simulink model "ap_12BAdapted"  (R2019b)
settings: Solver=FixedStepDiscrete  StartTime=0.0  StopTime=500  FixedStep=Ts  RelTol=1e-3  EnableMultiTasking=on
undefined symbols (not defined in the file): beaver_b, beaver_c, beaver_mass, beaver_S, Cl0, Cl_alpha2_dpt, Cl_beta, Cl_da, Cl_da_alpha, Cl_dr, Cl_p, Cl_r, Cm0, Cm_alpha, Cm_alpha2, Cm_beta2, Cm_de, Cm_df, Cm_dpt, Cm_q, Cm_r, Cn0, Cn_beta, Cn_beta3, Cn_da, Cn_dpt3, Cn_dr, Cn_p, Cn_q, Cn_r, Cx0, Cx_alpha, Cx_alpha2, Cx_alpha3, Cx_df, Cx_df_alpha, Cx_dpt, Cx_dpt2_alpha, Cx_dr, Cx_q, Cy0, Cy_beta, Cy_da, Cy_dr, Cy_dr_alpha, Cy_p, Cy_r, Cz0, Cz_alpha, Cz_alpha3, Cz_de, Cz_de_beta, Cz_df, Cz_df_alpha, Cz_dpt, Cz_q, d2r, fin_act_1, fin_act_2, fin_act_3 ... (+23)
libraries: simulink x10
(part 1 of 3)
settings Model: Creator=elliocm  LastModifiedBy=hbourbou
settings DataIOCC: LimitDataPoints=on  SaveFormat=Array  ReturnWorkspaceOutputs=off
settings OptimizationCC: ExpressionDepthLimit=2147483647  LifeSpan=inf
settings DebuggingCC: SolverPrmCheckMsg=warning  StateNameClashWarn=warning  SFUnexpectedBacktrackingDiag=warning  SFNoUnconditionalDefaultTransitionDiag=warning  SFExecutionAtInitializationDiag=none  ArithmeticOperatorsInVariantConditions=warning
settings HardwareCC: ProdBitPerPointer=32  ProdBitPerSizeT=32  ProdBitPerPtrDiffT=32  ProdLargestAtomicFloat=None  ProdIntDivRoundTo=Undefined  ProdEndianess=Unspecified  ProdWordSize=32  ProdHWDeviceType=32-bit Generic
settings ModelReferenceCC: PropagateSignalLabelsOutOfModel=off
settings SFSimCC: SimUseLocalCustomCode=off  CustomCodeUndefinedFunction=UseInterfaceOnly
settings RTWCC: RTWUseLocalCustomCode=off
settings CodeAppCC: StateflowObjectComments=on
settings GRTTargetCC: TargetLangStandard=C89/C90 (ANSI)  GeneratePreprocessorConditionals=Disable all
settings ConfigComp: CovMetricSettings=dw  CovHtmlReporting=on  CovSaveCumulativeToWorkspaceVar=on  CovSaveSingleToWorkspaceVar=on  CovExternalEMLEnable=off

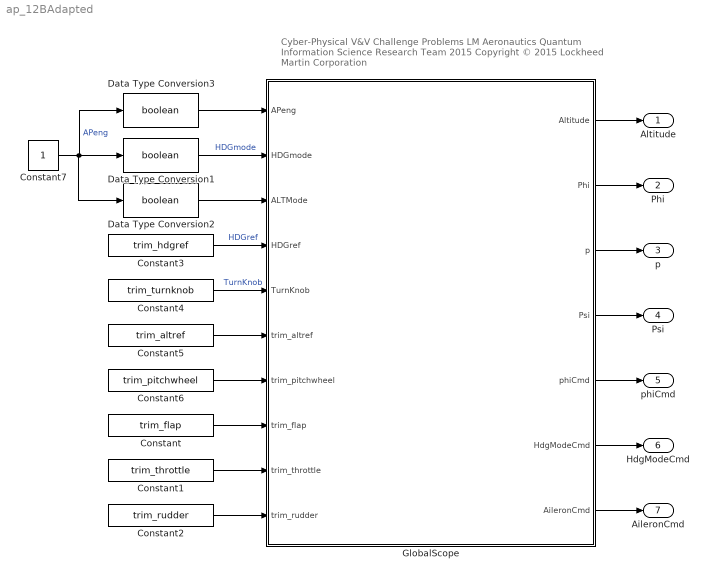
== system ap_12BAdapted ==
  note: Cyber-Physical V&V Challenge Problems
      | LM Aeronautics Quantum Information Science Research Team 2015
      | Copyright © 2015 Lockheed Martin Corporation
  Constant : Constant  Value=trim_flap
  Constant1 : Constant  Value=trim_throttle
  Constant2 : Constant  Value=trim_rudder
  Constant3 : Constant  Value=trim_hdgref
  Constant4 : Constant  Value=trim_turnknob
  Constant5 : Constant  Value=trim_altref
  Constant6 : Constant  Value=trim_pitchwheel
  Constant7 : Constant
  Data Type Conversion1 : DataTypeConversion  OutDataTypeStr=boolean
  Data Type Conversion2 : DataTypeConversion  OutDataTypeStr=boolean
  Data Type Conversion3 : DataTypeConversion  OutDataTypeStr=boolean
  GlobalScope : Subsystem
  Altitude : Outport  VectorParamsAs1DForOutWhenUnconnected=off
  Phi : Outport  Port=2  VectorParamsAs1DForOutWhenUnconnected=off
  p : Outport  Port=3  VectorParamsAs1DForOutWhenUnconnected=off
  Psi : Outport  Port=4  VectorParamsAs1DForOutWhenUnconnected=off
  phiCmd : Outport  Port=5  VectorParamsAs1DForOutWhenUnconnected=off
  HdgModeCmd : Outport  Port=6  VectorParamsAs1DForOutWhenUnconnected=off
  AileronCmd : Outport  Port=7  VectorParamsAs1DForOutWhenUnconnected=off
  wires:
  Constant7/1 -> Data Type Conversion2/1, Data Type Conversion3/1, Data Type Conversion1/1  "APeng"
  Data Type Conversion3/1 -> GlobalScope/1(APeng)
  Data Type Conversion1/1 -> GlobalScope/2(HDGmode)  "HDGmode"
  Data Type Conversion2/1 -> GlobalScope/3(ALTMode)
  Constant3/1 -> GlobalScope/4(HDGref)  "HDGref"
  Constant4/1 -> GlobalScope/5(TurnKnob)  "TurnKnob"
  Constant5/1 -> GlobalScope/6(trim_altref)
  Constant6/1 -> GlobalScope/7(trim_pitchwheel)
  GlobalScope/1(Altitude) -> Altitude/1
  Constant/1 -> GlobalScope/8(trim_flap)
  Constant2/1 -> GlobalScope/10(trim_rudder)
  Constant1/1 -> GlobalScope/9(trim_throttle)
  GlobalScope/6(HdgModeCmd) -> HdgModeCmd/1
  GlobalScope/5(phiCmd) -> phiCmd/1
  GlobalScope/7(AileronCmd) -> AileronCmd/1
  GlobalScope/4(Psi) -> Psi/1
  GlobalScope/3(p) -> p/1
  GlobalScope/2(Phi) -> Phi/1

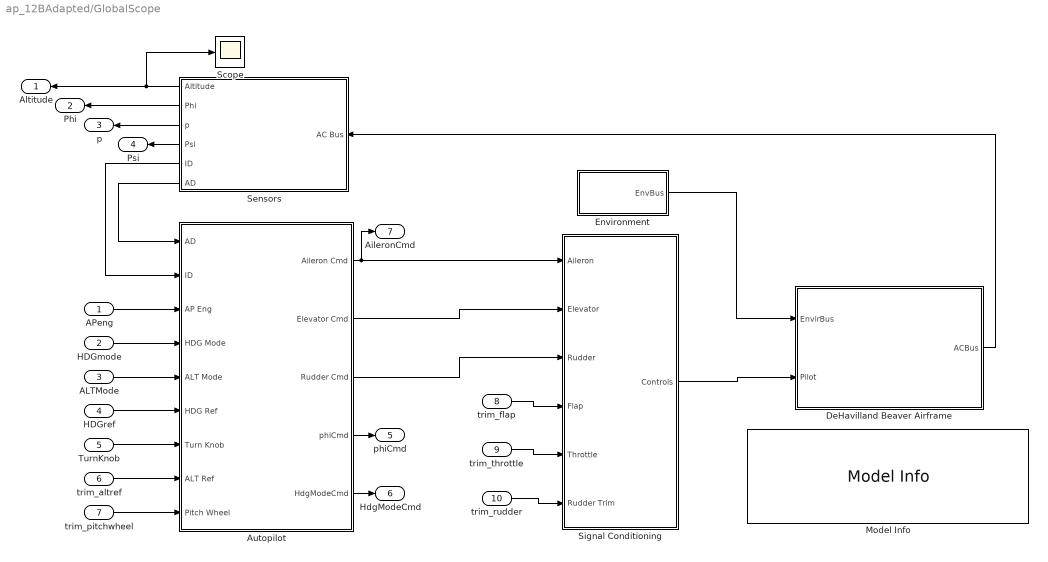
== system ap_12BAdapted/GlobalScope ==
  APeng : Inport
  HDGmode : Inport  Port=2
  ALTMode : Inport  Port=3
  HDGref : Inport  Port=4
  TurnKnob : Inport  Port=5
  trim_altref : Inport  Port=6
  trim_pitchwheel : Inport  Port=7
  trim_flap : Inport  Port=8
  trim_throttle : Inport  Port=9
  trim_rudder : Inport  Port=10
  Autopilot : Subsystem  TreatAsAtomicUnit=on
  DeHavilland Beaver Airframe : Subsystem  TreatAsAtomicUnit=on
      mask Display:
      | %image(imread('asbbeaver.jpg'))
      | image(imread('asbbeaver.png'))
  Environment : Subsystem
  Model Info : simulink/Model-Wide Utilities/Model Info  Frame=on  DisplayStringWithTags=|  HorizontalTextAlignment=Center  LeftAlignmentValue=0.5
      | DeHavilland Beaver model 
      | originally based on work created by
      | Marc Rauw for Delft University of Technology,  
      | http://www.dutchroll.com
      | and subsequently modified by the Mathworks
      | http://www.mathworks.com/matlabcentral/fileexchange/
  Scope : Scope
  Sensors : Subsystem
  Signal Conditioning : Subsystem  TreatAsAtomicUnit=on
  Altitude : Outport  VectorParamsAs1DForOutWhenUnconnected=off
  Phi : Outport  Port=2  VectorParamsAs1DForOutWhenUnconnected=off
  p : Outport  Port=3  VectorParamsAs1DForOutWhenUnconnected=off
  Psi : Outport  Port=4  VectorParamsAs1DForOutWhenUnconnected=off
  phiCmd : Outport  Port=5  VectorParamsAs1DForOutWhenUnconnected=off
  HdgModeCmd : Outport  Port=6  VectorParamsAs1DForOutWhenUnconnected=off
  AileronCmd : Outport  Port=7  VectorParamsAs1DForOutWhenUnconnected=off
  wires:
  Autopilot/1(Aileron Cmd) -> AileronCmd/1, Signal Conditioning/1(Aileron)
  Sensors/1(Altitude) -> Altitude/1, Scope/1
  trim_altref/1 -> Autopilot/8(ALT Ref)
  Autopilot/3(Rudder Cmd) -> Signal Conditioning/3(Rudder)
  ALTMode/1 -> Autopilot/5(ALT Mode)
  TurnKnob/1 -> Autopilot/7(Turn Knob)
  trim_throttle/1 -> Signal Conditioning/5(Throttle)
  trim_rudder/1 -> Signal Conditioning/6(Rudder Trim)
  trim_flap/1 -> Signal Conditioning/4(Flap)
  trim_pitchwheel/1 -> Autopilot/9(Pitch Wheel)
  APeng/1 -> Autopilot/3(AP Eng)
  Environment/1(EnvBus) -> DeHavilland Beaver Airframe/1(EnvirBus)
  Autopilot/2(Elevator Cmd) -> Signal Conditioning/2(Elevator)
  DeHavilland Beaver Airframe/1(ACBus) -> Sensors/1(AC Bus)
  HDGmode/1 -> Autopilot/4(HDG Mode)
  HDGref/1 -> Autopilot/6(HDG Ref)
  Sensors/6(AD) -> Autopilot/1(AD)
  Sensors/5(ID) -> Autopilot/2(ID)
  Autopilot/4(phiCmd) -> phiCmd/1
  Sensors/2(Phi) -> Phi/1
  Sensors/3(p) -> p/1
  Autopilot/5(HdgModeCmd) -> HdgModeCmd/1
  Sensors/4(Psi) -> Psi/1
  Signal Conditioning/1(Controls) -> DeHavilland Beaver Airframe/2(Pilot)

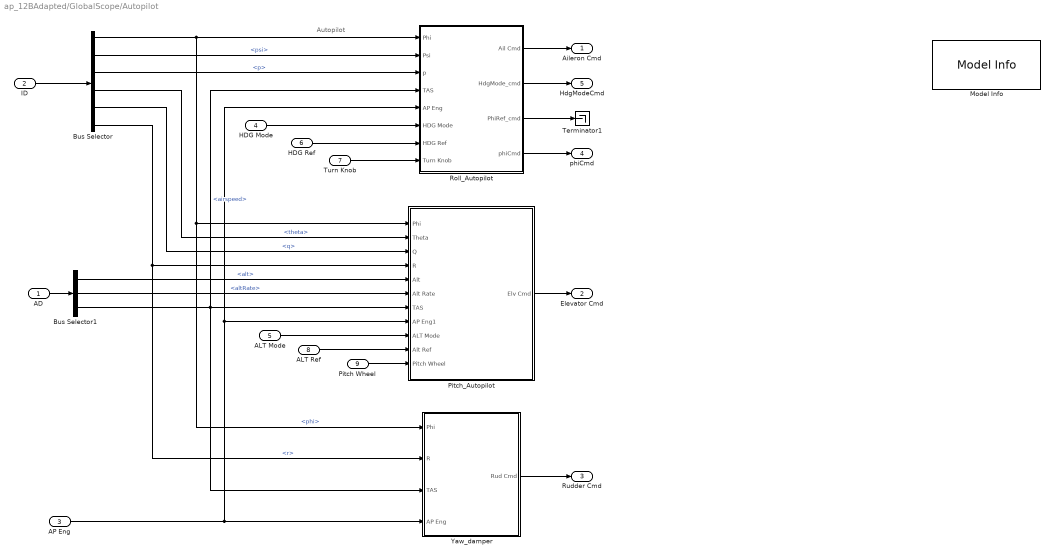
== system ap_12BAdapted/GlobalScope/Autopilot ==
  note: Autopilot
  AD : Inport
  ID : Inport  Port=2
  AP Eng : Inport  Port=3  OutMin=0  OutMax=1  OutDataTypeStr=boolean  PortDimensions=1
  HDG Mode : Inport  Port=4  OutMin=0  OutMax=1  OutDataTypeStr=boolean  PortDimensions=1
  ALT Mode : Inport  Port=5  OutMin=0  OutMax=1  OutDataTypeStr=boolean  PortDimensions=1
  HDG Ref : Inport  Port=6  OutMin=-180  OutMax=180  OutDataTypeStr=double  PortDimensions=1
  Turn Knob : Inport  Port=7  OutMin=-45  OutMax=45  OutDataTypeStr=double  PortDimensions=1
  ALT Ref : Inport  Port=8  OutMin=0  OutMax=65000  OutDataTypeStr=double  PortDimensions=1
  Pitch Wheel : Inport  Port=9  OutMin=-30  OutMax=30  OutDataTypeStr=double  PortDimensions=1
  Bus Selector : BusSelector  OutputSignals=phi,psi,p,theta,q,r
  Bus Selector1 : BusSelector  OutputSignals=alt,altRate,airspeed
  Model Info : simulink/Model-Wide Utilities/Model Info  Frame=on  DisplayStringWithTags=|  HorizontalTextAlignment=Left  LeftAlignmentValue=0.02
      | Autopilot
      | Author: %<LastModifiedBy>
      | Date: %<LastModificationDate>
      | Model Version: %<ModelVersion>
  Pitch_Autopilot : Subsystem
  Roll_Autopilot : Subsystem
  Terminator1 : Terminator
  Yaw_damper : Subsystem
  Aileron Cmd : Outport  OutDataTypeStr=double  PortDimensions=1  SampleTime=[0.025000000000000001,0]  VectorParamsAs1DForOutWhenUnconnected=off
  Elevator Cmd : Outport  Port=2  OutDataTypeStr=double  PortDimensions=1  SampleTime=[0.025000000000000001,0]  VectorParamsAs1DForOutWhenUnconnected=off
  Rudder Cmd : Outport  Port=3  OutDataTypeStr=double  PortDimensions=1  SampleTime=[0.025000000000000001,0]  VectorParamsAs1DForOutWhenUnconnected=off
  phiCmd : Outport  Port=4  VectorParamsAs1DForOutWhenUnconnected=off
  HdgModeCmd : Outport  Port=5  VectorParamsAs1DForOutWhenUnconnected=off
  wires:
  Roll_Autopilot/1(Ail Cmd) -> Aileron Cmd/1
  HDG Ref/1 -> Roll_Autopilot/7(HDG Ref)
  Bus Selector/6 -> Yaw_damper/2(R), Pitch_Autopilot/4(R)  "<r>"
  Bus Selector1/3 -> Yaw_damper/3(TAS), Roll_Autopilot/4(TAS), Pitch_Autopilot/7(TAS)  "<airspeed>"
  HDG Mode/1 -> Roll_Autopilot/6(HDG Mode)
  Pitch_Autopilot/1(Elv Cmd) -> Elevator Cmd/1
  ALT Mode/1 -> Pitch_Autopilot/9(ALT Mode)
  ALT Ref/1 -> Pitch_Autopilot/10(Alt Ref)
  Pitch Wheel/1 -> Pitch_Autopilot/11("Pitch Wheel ")
  Bus Selector1/1 -> Pitch_Autopilot/5(Alt)  "<alt>"
  Yaw_damper/1(Rud Cmd) -> Rudder Cmd/1
  AP Eng/1 -> Yaw_damper/4(AP Eng), Roll_Autopilot/5(AP Eng), Pitch_Autopilot/8(AP Eng1)
  Bus Selector/3 -> Roll_Autopilot/3(p)  "<p>"
  Turn Knob/1 -> Roll_Autopilot/8(Turn Knob)
  Bus Selector/1 -> Pitch_Autopilot/1(Phi), Yaw_damper/1(Phi), Roll_Autopilot/1(Phi)  "<phi>"
  Bus Selector/2 -> Roll_Autopilot/2(Psi)  "<psi>"
  Bus Selector/5 -> Pitch_Autopilot/3(Q)  "<q>"
  Bus Selector/4 -> Pitch_Autopilot/2(Theta)  "<theta>"
  ID/1 -> Bus Selector/1
  AD/1 -> Bus Selector1/1
  Bus Selector1/2 -> Pitch_Autopilot/6(Alt Rate)  "<altRate>"
  Roll_Autopilot/4(phiCmd) -> phiCmd/1
  Roll_Autopilot/2(HdgMode_cmd) -> HdgModeCmd/1
  Roll_Autopilot/3(PhiRef_cmd) -> Terminator1/1

== system ap_12BAdapted/GlobalScope/DeHavilland Beaver Airframe ==
  note: DeHavilland Beaver Airframe
  EnvirBus : Inport
  Pilot : Inport  Port=2
  Aircraft Dynamics : Subsystem
  Calculate Parameters : Subsystem
  ACBus : Outport  VectorParamsAs1DForOutWhenUnconnected=off
  wires:
  Pilot/1 -> Aircraft Dynamics/1(Pilot)
  Aircraft Dynamics/1(AC Bus) -> ACBus/1, Calculate Parameters/2(ACBus)
  EnvirBus/1 -> Aircraft Dynamics/2(EnvirBus), Calculate Parameters/1(EnvirBus)
  Calculate Parameters/1(FltParams) -> Aircraft Dynamics/3(FltParams)

== system ap_12BAdapted/GlobalScope/Environment ==
  note: Environment
  Bus Creator : BusCreator  Inputs=3
  Bus Creator1 : BusCreator  Inputs=2
  Mux : Mux  Inputs=3
  Mux1 : Mux  Inputs=3
  g_mps2 : Constant  Value=9.799
  rho_kgpm3 : Constant  Value=0.9862
  wind_mps : Constant  Value=0
  EnvBus : Outport  VectorParamsAs1DForOutWhenUnconnected=off
  wires:
  g_mps2/1 -> Bus Creator/1  "g"
  Mux1/1 -> Bus Creator1/2  "pqr_wind"
  Mux/1 -> Bus Creator1/1  "uvw_wind"
  Bus Creator1/1 -> Bus Creator/3  "Vwind"
  Bus Creator/1 -> EnvBus/1
  rho_kgpm3/1 -> Bus Creator/2  "rho"
  wind_mps/1 -> Mux1/3, Mux1/2, Mux1/1, Mux/3, Mux/2, Mux/1

== system ap_12BAdapted/GlobalScope/Sensors ==
  AC Bus : Inport
  Air Data Sensor : Subsystem
  Bus Creator : BusCreator  Inputs=6
  Bus Creator1 : BusCreator  Inputs=5
  Bus Creator2 : BusCreator  Inputs=2
  Display : Display
  Display1 : Display
  Inertial Data Sensor : Subsystem
  Scope : Scope  NumInputPorts=5
  Scope1 : Scope  NumInputPorts=6
  Terminator : Terminator
  Altitude : Outport  VectorParamsAs1DForOutWhenUnconnected=off
  Phi : Outport  Port=2  VectorParamsAs1DForOutWhenUnconnected=off
  p : Outport  Port=3  VectorParamsAs1DForOutWhenUnconnected=off
  Psi : Outport  Port=4  VectorParamsAs1DForOutWhenUnconnected=off
  ID : Outport  Port=5  VectorParamsAs1DForOutWhenUnconnected=off
  AD : Outport  Port=6  VectorParamsAs1DForOutWhenUnconnected=off
  wires:
  AC Bus/1 -> Air Data Sensor/1(AC Bus), Inertial Data Sensor/1(AC Bus)
  Inertial Data Sensor/3(psi) -> Scope1/3, Psi/1, Bus Creator/3  "psi"
  Inertial Data Sensor/2(theta) -> Scope1/2, Bus Creator/2  "theta"
  Inertial Data Sensor/4(p) -> Scope1/4, p/1, Bus Creator/4  "p"
  Inertial Data Sensor/1(phi) -> Scope1/1, Phi/1, Bus Creator/1
  Inertial Data Sensor/5(q) -> Scope1/5, Bus Creator/5  "q"
  Inertial Data Sensor/6(r) -> Scope1/6, Bus Creator/6  "r"
  Bus Creator/1 -> Bus Creator2/1, Display/1, ID/1  "ID"
  Air Data Sensor/1(altRate) -> Scope/1, Bus Creator1/1  "altRate"
  Air Data Sensor/2(alpha) -> Scope/2, Bus Creator1/2  "alpha"
  Air Data Sensor/3(beta) -> Scope/3, Bus Creator1/3  "beta"
  Air Data Sensor/4(airspeed) -> Scope/4, Bus Creator1/4  "airspeed"
  Air Data Sensor/5(alt) -> Scope/5, Altitude/1, Bus Creator1/5  "alt"
  Bus Creator1/1 -> Bus Creator2/2, Display1/1, AD/1  "AD"
  Bus Creator2/1 -> Terminator/1

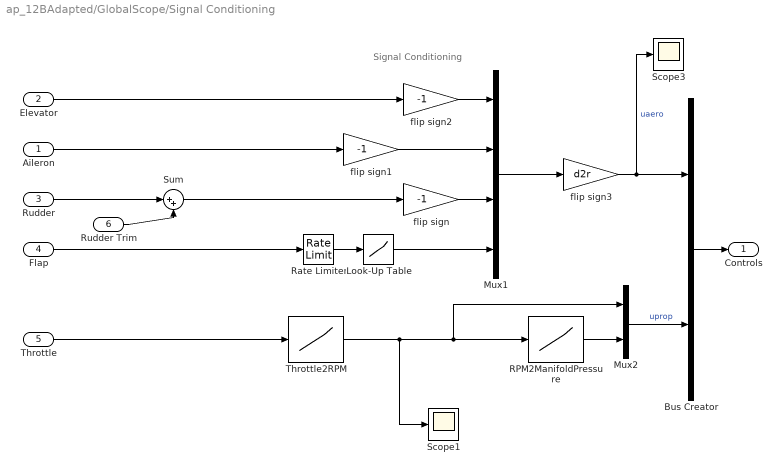
== system ap_12BAdapted/GlobalScope/Signal Conditioning ==
  note: Signal Conditioning
  Aileron : Inport
  Elevator : Inport  Port=2
  Rudder : Inport  Port=3
  Flap : Inport  Port=4
  Throttle : Inport  Port=5
  Rudder Trim : Inport  Port=6
  Bus Creator : BusCreator  Inputs=2
  Look-Up Table : Lookup_n-D  NumberOfTableDimensions=1  BreakpointsForDimension1=[0:3]  Table=[0 4 10 20]  InternalRulePriority=Speed  SaturateOnIntegerOverflow=on  InputSameDT=on
  Mux1 : Mux
  Mux2 : Mux  Inputs=2
  RPM2ManifoldPressure : Lookup_n-D  NumberOfTableDimensions=1  BreakpointsForDimension1=[0 1800 2300]  IndexSearchMethod=Linear search  BeginIndexSearchUsingPreviousIndexResult=on  Table=[0 22.5735 26]  ExtrapMethod=Clip  InputSameDT=on
  Rate Limiter : RateLimiter  RisingSlewLimit=0.5  FallingSlewLimit=-0.5
  Scope1 : Scope
  Scope3 : Scope
  Sum : Sum  Inputs=|++
  Throttle2RPM : Lookup_n-D  NumberOfTableDimensions=1  BreakpointsForDimension1=(1/6)*(3+([-3:3]))  IndexSearchMethod=Linear search  BeginIndexSearchUsingPreviousIndexResult=on  Table=((1+tanh([-3:3]))/(1+tanh(2.65))-0.0025)*2300  ExtrapMethod=Clip  InputSameDT=on
  flip sign : Gain  Gain=-1  SaturateOnIntegerOverflow=on  OutDataTypeStr=Inherit: Same as input  ParamDataTypeStr=Inherit: Same as input
  flip sign1 : Gain  Gain=-1  SaturateOnIntegerOverflow=on  OutDataTypeStr=Inherit: Same as input  ParamDataTypeStr=Inherit: Same as input
  flip sign2 : Gain  Gain=-1  SaturateOnIntegerOverflow=on  OutDataTypeStr=Inherit: Same as input  ParamDataTypeStr=Inherit: Same as input
  flip sign3 : Gain  Gain=d2r  SaturateOnIntegerOverflow=on  OutDataTypeStr=Inherit: Same as input  ParamDataTypeStr=Inherit: Same as input
  Controls : Outport  VectorParamsAs1DForOutWhenUnconnected=off
  wires:
  Bus Creator/1 -> Controls/1
  Throttle/1 -> Throttle2RPM/1
  Sum/1 -> flip sign/1
  Aileron/1 -> flip sign1/1
  Elevator/1 -> flip sign2/1
  flip sign2/1 -> Mux1/1
  flip sign1/1 -> Mux1/2
  Throttle2RPM/1 -> Scope1/1, RPM2ManifoldPressure/1, Mux2/1
  flip sign/1 -> Mux1/3
  Mux2/1 -> Bus Creator/2  "uprop"
  RPM2ManifoldPressure/1 -> Mux2/2
  flip sign3/1 -> Scope3/1, Bus Creator/1  "uaero"
  Mux1/1 -> flip sign3/1
  Look-Up Table/1 -> Mux1/4
  Rate Limiter/1 -> Look-Up Table/1
  Rudder/1 -> Sum/1
  Rudder Trim/1 -> Sum/2
  Flap/1 -> Rate Limiter/1

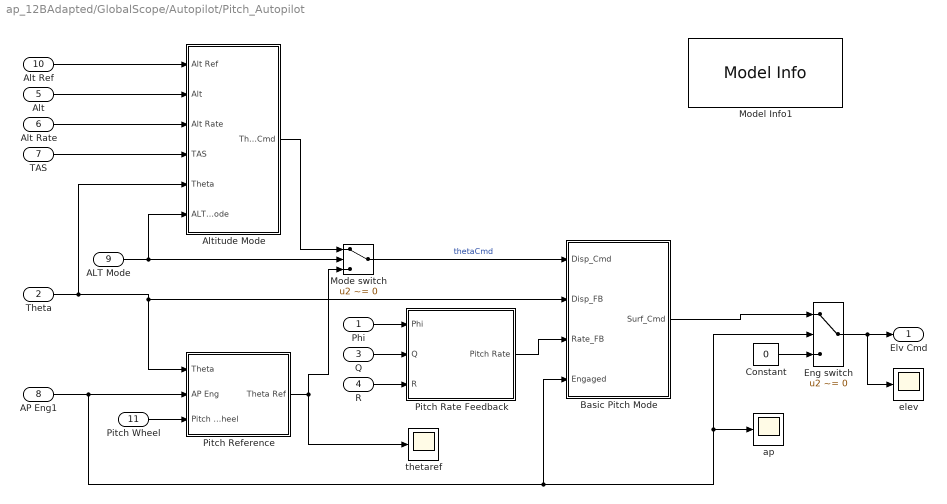
== system ap_12BAdapted/GlobalScope/Autopilot/Pitch_Autopilot ==
  Phi : Inport  OutDataTypeStr=double  PortDimensions=1  SampleTime=1/40  Interpolate=off
  Theta : Inport  Port=2  OutDataTypeStr=double  PortDimensions=1  SampleTime=1/40  Interpolate=off
  Q : Inport  Port=3  OutDataTypeStr=double  PortDimensions=1  SampleTime=1/40  Interpolate=off
  R : Inport  Port=4  OutDataTypeStr=double  PortDimensions=1  SampleTime=1/40  Interpolate=off
  Alt : Inport  Port=5  OutDataTypeStr=double  PortDimensions=1  SampleTime=1/40  Interpolate=off
  Alt Rate : Inport  Port=6  OutDataTypeStr=double  PortDimensions=1  SampleTime=1/40  Interpolate=off
  TAS : Inport  Port=7  OutDataTypeStr=double  PortDimensions=1  SampleTime=1/40  Interpolate=off
  AP Eng1 : Inport  Port=8  OutDataTypeStr=boolean  PortDimensions=1  SampleTime=1/40  Interpolate=off
  ALT Mode : Inport  Port=9  OutDataTypeStr=boolean  PortDimensions=1  SampleTime=1/40  Interpolate=off
  Alt Ref : Inport  Port=10  OutDataTypeStr=double  PortDimensions=1  SampleTime=1/40  Interpolate=off
  "Pitch Wheel " : Inport  Port=11  OutDataTypeStr=double  PortDimensions=1  SampleTime=1/40  Interpolate=off
  Altitude Mode : Subsystem
  Basic Pitch Mode : Subsystem
  Constant : Constant  Value=0  OutDataTypeStr=double
  Eng switch : Switch  Criteria=u2 ~= 0
  Mode switch : Switch  Criteria=u2 ~= 0
  Model Info1 : simulink/Model-Wide Utilities/Model Info  Frame=on  DisplayStringWithTags=|  HorizontalTextAlignment=Left  LeftAlignmentValue=0.02
      | Pitch Autopilot
      | Author: %<LastModifiedBy>
      | Date: %<LastModificationDate>
      | Model Version: %<ModelVersion>
  Pitch Rate Feedback : Subsystem  TreatAsAtomicUnit=on
      settings: RTWSystemCode=Inline
  Pitch Reference : Subsystem  TreatAsAtomicUnit=on
      settings: RTWSystemCode=Inline
  ap : Scope
  elev : Scope
  thetaref : Scope
  Elv Cmd : Outport  OutDataTypeStr=double  PortDimensions=1  SampleTime=1/40  VectorParamsAs1DForOutWhenUnconnected=off
  wires:
  "Pitch Wheel "/1 -> Pitch Reference/3(Pitch Wheel)
  Pitch Rate Feedback/1(Pitch Rate) -> Basic Pitch Mode/3(Rate_FB)
  Alt Ref/1 -> Altitude Mode/1(Alt Ref)
  Theta/1 -> Altitude Mode/5(Theta), Pitch Reference/1(Theta), Basic Pitch Mode/2("Disp_FB ")
  Q/1 -> Pitch Rate Feedback/2(Q)
  Eng switch/1 -> elev/1, Elv Cmd/1
  Constant/1 -> Eng switch/3
  Phi/1 -> Pitch Rate Feedback/1(Phi)
  R/1 -> Pitch Rate Feedback/3(R)
  TAS/1 -> Altitude Mode/4(TAS)
  Pitch Reference/1(Theta Ref) -> thetaref/1, Mode switch/3
  Alt/1 -> Altitude Mode/2(Alt)
  Alt Rate/1 -> Altitude Mode/3(Alt Rate)
  Mode switch/1 -> Basic Pitch Mode/1(Disp_Cmd)  "thetaCmd"
  ALT Mode/1 -> Altitude Mode/6(ALT Mode), Mode switch/2
  Altitude Mode/1(Theta Cmd) -> Mode switch/1
  AP Eng1/1 -> Eng switch/2, ap/1, Basic Pitch Mode/4(Engaged), Pitch Reference/2(AP Eng)
  Basic Pitch Mode/1(Surf_Cmd) -> Eng switch/1

== system ap_12BAdapted/GlobalScope/Autopilot/Roll_Autopilot ==
  Phi : Inport  OutMin=-180  OutMax=180  OutDataTypeStr=double  PortDimensions=1  SampleTime=1/40  Interpolate=off
  Psi : Inport  Port=2  OutMin=-180  OutMax=180  OutDataTypeStr=double  PortDimensions=1  SampleTime=1/40  Interpolate=off
  p : Inport  Port=3  OutMin=-180  OutMax=180  OutDataTypeStr=double  PortDimensions=1  Interpolate=off
  TAS : Inport  Port=4  OutMin=0  OutMax=1000  OutDataTypeStr=double  PortDimensions=1  SampleTime=1/40  Interpolate=off
  AP Eng : Inport  Port=5  OutDataTypeStr=boolean  PortDimensions=1  SampleTime=1/40  Interpolate=off
  HDG Mode : Inport  Port=6  OutDataTypeStr=boolean  PortDimensions=1  SampleTime=1/40  Interpolate=off
  HDG Ref : Inport  Port=7  OutMin=-180  OutMax=180  OutDataTypeStr=double  PortDimensions=1  SampleTime=1/40  Interpolate=off
  Turn Knob : Inport  Port=8  OutMin=-45  OutMax=45  OutDataTypeStr=double  PortDimensions=1  SampleTime=1/40  Interpolate=off
  Basic Roll Mode : Subsystem
  Eng switch : Switch  Criteria=u2 ~= 0
  Heading Mode : Subsystem
  Mode switch : Switch  Criteria=u2 ~= 0
  Roll Reference : Subsystem  TreatAsAtomicUnit=on
      settings: RTWSystemCode=Inline
  Scope1 : Scope
  zero : Constant  Value=0  OutDataTypeStr=double
  Ail Cmd : Outport  OutDataTypeStr=double  PortDimensions=1  SampleTime=1/40  VectorParamsAs1DForOutWhenUnconnected=off
  HdgMode_cmd : Outport  Port=2  VectorParamsAs1DForOutWhenUnconnected=off
  PhiRef_cmd : Outport  Port=3  VectorParamsAs1DForOutWhenUnconnected=off
  phiCmd : Outport  Port=4  VectorParamsAs1DForOutWhenUnconnected=off
  wires:
  HDG Ref/1 -> Heading Mode/1(Psi Ref)
  Heading Mode/1(Phi Cmd) -> HdgMode_cmd/1, Mode switch/1
  Mode switch/1 -> phiCmd/1, Basic Roll Mode/1(Disp_Cmd)  "phiCmd"
  Eng switch/1 -> Ail Cmd/1
  AP Eng/1 -> Roll Reference/2(AP eng), Basic Roll Mode/4(Engaged), Eng switch/2
  TAS/1 -> Heading Mode/3(TAS)
  HDG Mode/1 -> Mode switch/2
  Roll Reference/1(Phi Ref) -> Mode switch/3, PhiRef_cmd/1
  Turn Knob/1 -> Roll Reference/3(Turn Knob)
  zero/1 -> Eng switch/3
  p/1 -> Basic Roll Mode/3(Rate_FB)
  Phi/1 -> Scope1/1, Basic Roll Mode/2("Disp_FB "), Roll Reference/1(Phi)
  Psi/1 -> Heading Mode/2(Psi)
  Basic Roll Mode/1(Surf_Cmd) -> Eng switch/1

== system ap_12BAdapted/GlobalScope/Autopilot/Yaw_damper ==
  Phi : Inport  OutDataTypeStr=double  PortDimensions=1  SampleTime=1/40  Interpolate=off
  R : Inport  Port=2  OutDataTypeStr=double  PortDimensions=1  SampleTime=1/40  Interpolate=off
  TAS : Inport  Port=3  OutDataTypeStr=double  PortDimensions=1  SampleTime=1/40  Interpolate=off
  AP Eng : Inport  Port=4  OutDataTypeStr=boolean  PortDimensions=1  SampleTime=1/40  Interpolate=off
  Basic Yaw Damper : Subsystem  TreatAsAtomicUnit=on
      settings: RTWSystemCode=Inline
  Constant : Constant  Value=0  OutDataTypeStr=double
  Eng switch : Switch  Criteria=u2 ~= 0
  Model Info1 : simulink/Model-Wide Utilities/Model Info  Frame=on  DisplayStringWithTags=|  HorizontalTextAlignment=Left  LeftAlignmentValue=0.02
      | Yaw Damper
      | Author: %<LastModifiedBy>
      | Version: %<ModelVersion>
      | Date: %<LastModificationDate>
  Rud Cmd : Outport  OutDataTypeStr=double  PortDimensions=1  SampleTime=1/40  VectorParamsAs1DForOutWhenUnconnected=off
  wires:
  Phi/1 -> Basic Yaw Damper/1("Phi ")
  R/1 -> Basic Yaw Damper/2(R)
  Constant/1 -> Eng switch/3
  TAS/1 -> Basic Yaw Damper/3(TAS)
  Basic Yaw Damper/1(Rud Cmd) -> Eng switch/1
  Eng switch/1 -> Rud Cmd/1
  AP Eng/1 -> Eng switch/2

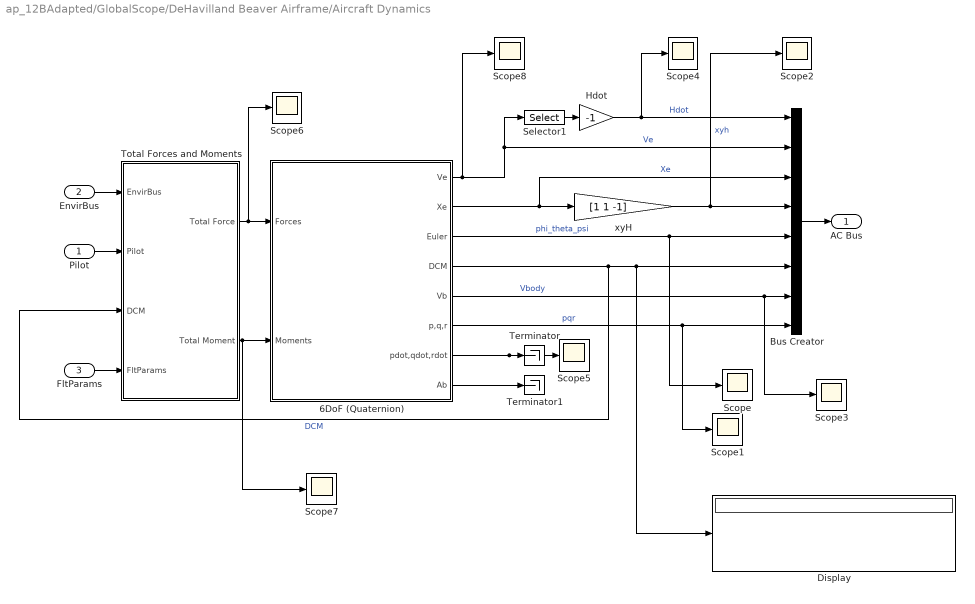
== system ap_12BAdapted/GlobalScope/DeHavilland Beaver Airframe/Aircraft Dynamics ==
  Pilot : Inport
  EnvirBus : Inport  Port=2
  FltParams : Inport  Port=3
  6DoF (Quaternion) : Subsystem
  Bus Creator : BusCreator  Inputs=8
  Display : Display
  Hdot : Gain  Gain=-1  SaturateOnIntegerOverflow=on  OutDataTypeStr=Inherit: Same as input  ParamDataTypeStr=Inherit: Same as input
  Scope{,1..8} (9 alike) : Scope
  Selector1 : Selector  InputPortWidth=3  IndexOptions=Index vector (dialog)  Indices=[3]  OutputSizes=1
  Terminator : Terminator
  Terminator1 : Terminator
  Total Forces and Moments : Subsystem
  xyH : Gain  Gain=[1 1 -1]  SaturateOnIntegerOverflow=on  OutDataTypeStr=Inherit: Same as input  ParamDataTypeStr=Inherit: Same as input
  AC Bus : Outport  VectorParamsAs1DForOutWhenUnconnected=off
  wires:
  6DoF (Quaternion)/4(DCM) -> Display/1, Bus Creator/6, Total Forces and Moments/3(DCM)  "DCM"
  6DoF (Quaternion)/3(Euler) -> Scope/1, Bus Creator/5  "phi_theta_psi"
  6DoF (Quaternion)/2(Xe) -> xyH/1, Bus Creator/3  "Xe"
  6DoF (Quaternion)/5(Vb) -> Scope3/1, Bus Creator/7  "Vbody"
  6DoF (Quaternion)/7(pdot,qdot,rdot) -> Scope5/1, Terminator/1
  6DoF (Quaternion)/1(Ve) -> Scope8/1, Selector1/1, Bus Creator/2  "Ve"
  Pilot/1 -> Total Forces and Moments/2(Pilot)
  Selector1/1 -> Hdot/1
  Total Forces and Moments/1(Total Force) -> Scope6/1, 6DoF (Quaternion)/1(Forces)
  Total Forces and Moments/2(Total Moment) -> Scope7/1, 6DoF (Quaternion)/2(Moments)
  xyH/1 -> Scope2/1, Bus Creator/4  "xyh"
  Hdot/1 -> Scope4/1, Bus Creator/1  "Hdot"
  6DoF (Quaternion)/8(Ab) -> Terminator1/1
  Bus Creator/1 -> AC Bus/1
  EnvirBus/1 -> Total Forces and Moments/1(EnvirBus)
  6DoF (Quaternion)/6(p,q,r) -> Scope1/1, Bus Creator/8  "pqr"
  FltParams/1 -> Total Forces and Moments/4(FltParams)

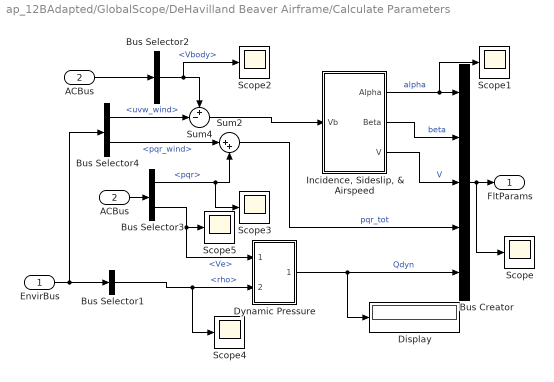
== system ap_12BAdapted/GlobalScope/DeHavilland Beaver Airframe/Calculate Parameters ==
  EnvirBus : Inport
  ACBus : Inport  Port=2
  " Incidence, Sideslip, & Airspeed" : Subsystem
  "ACBus " : InportShadow  Port=2
  Bus Creator : BusCreator  Inputs=5
  Bus Selector1 : BusSelector  OutputSignals=rho
  Bus Selector2 : BusSelector  OutputSignals=Vbody
  Bus Selector3 : BusSelector  OutputSignals=pqr,Ve
  Bus Selector4 : BusSelector  OutputSignals=Vwind.uvw_wind,Vwind.pqr_wind
  Display : Display
  Dynamic Pressure : Subsystem
  Scope{,1..5} (6 alike) : Scope
  Sum2 : Sum  Inputs=|++  SaturateOnIntegerOverflow=on  InputSameDT=on  OutDataTypeStr=Inherit: Same as first input
  Sum4 : Sum  Inputs=+-|  SaturateOnIntegerOverflow=on  InputSameDT=on  OutDataTypeStr=Inherit: Same as first input
  FltParams : Outport  VectorParamsAs1DForOutWhenUnconnected=off
  wires:
  "ACBus "/1 -> Bus Selector2/1
  Bus Creator/1 -> Scope/1, FltParams/1
  Bus Selector3/1 -> Scope3/1, Sum2/2  "<pqr>"
  ACBus/1 -> Bus Selector3/1
  Bus Selector1/1 -> Scope4/1, Dynamic Pressure/2(Air Density)  "<rho>"
  EnvirBus/1 -> Bus Selector1/1, Bus Selector4/1
  Dynamic Pressure/1(qbar) -> Display/1, Bus Creator/5  "Qdyn"
  Bus Selector3/2 -> Scope5/1, Dynamic Pressure/1(Velocity)  "<Ve>"
  Bus Selector4/2 -> Sum2/1  "<pqr_wind>"
  Sum4/1 -> " Incidence, Sideslip, & Airspeed"/1(Vb)
  " Incidence, Sideslip, & Airspeed"/1(Alpha) -> Scope1/1, Bus Creator/1  "alpha"
  " Incidence, Sideslip, & Airspeed"/2(Beta) -> Bus Creator/2  "beta"
  " Incidence, Sideslip, & Airspeed"/3(V) -> Bus Creator/3  "V"
  Bus Selector2/1 -> Scope2/1, Sum4/1  "<Vbody>"
  Bus Selector4/1 -> Sum4/2  "<uvw_wind>"
  Sum2/1 -> Bus Creator/4  "pqr_tot"

== system ap_12BAdapted/GlobalScope/Sensors/Air Data Sensor ==
  note: Air Data Sensor
  AC Bus : Inport
  " Incidence, Sideslip, & Airspeed" : Subsystem
  Bus Selector1 : BusSelector  OutputSignals=Hdot,Vbody,xyh
  Constant1 : Constant  Value=trim_v
  Constant2 : Constant  Value=0.0
  Constant3 : Constant  Value=trim_altref
  Selector1 : Selector  InputPortWidth=3  IndexOptions=Index vector (dialog)  Indices=[3]  OutputSizes=1
  flip sign1 : Gain  Gain=m2ft  SaturateOnIntegerOverflow=on  OutDataTypeStr=Inherit: Same as input  ParamDataTypeStr=Inherit: Same as input
  flip sign2 : Gain  Gain=m2ft  SaturateOnIntegerOverflow=on  OutDataTypeStr=Inherit: Same as input  ParamDataTypeStr=Inherit: Same as input
  flip sign3 : Gain  Gain=m2ft  SaturateOnIntegerOverflow=on  OutDataTypeStr=Inherit: Same as input  ParamDataTypeStr=Inherit: Same as input
  ic1 : Subsystem
  ic2 : Subsystem
  ic3 : Subsystem
  altRate : Outport  VectorParamsAs1DForOutWhenUnconnected=off
  alpha : Outport  Port=2  VectorParamsAs1DForOutWhenUnconnected=off
  beta : Outport  Port=3  VectorParamsAs1DForOutWhenUnconnected=off
  airspeed : Outport  Port=4  VectorParamsAs1DForOutWhenUnconnected=off
  alt : Outport  Port=5  VectorParamsAs1DForOutWhenUnconnected=off
  wires:
  Constant1/1 -> ic1/2(ic)
  AC Bus/1 -> Bus Selector1/1
  flip sign3/1 -> ic2/1(u)  "alt"
  " Incidence, Sideslip, & Airspeed"/2(Beta) -> beta/1  "beta"
  Selector1/1 -> flip sign3/1
  ic1/1(y) -> flip sign1/1
  Constant3/1 -> ic2/2(ic)
  Constant2/1 -> ic3/2(ic)
  Bus Selector1/2 -> ic1/1(u)  "<Vbody>"
  " Incidence, Sideslip, & Airspeed"/3(V) -> airspeed/1  "airspeed"
  " Incidence, Sideslip, & Airspeed"/1(Alpha) -> alpha/1  "alpha"
  Bus Selector1/3 -> Selector1/1  "<xyh>"
  flip sign2/1 -> ic3/1(u)  "Hdotfps"
  ic2/1(y) -> alt/1  "alt"
  Bus Selector1/1 -> flip sign2/1  "<Hdot>"
  ic3/1(y) -> altRate/1  "altRate"
  flip sign1/1 -> " Incidence, Sideslip, & Airspeed"/1(Vb)  "Vfps"

== system ap_12BAdapted/GlobalScope/Sensors/Inertial Data Sensor ==
  note: Inertial Data Sensor
  AC Bus : Inport
  Bus Selector : BusSelector  OutputSignals=phi_theta_psi,pqr
  Constant : Constant  Value=0.0
  Constant1 : Constant  Value=trim_hdg
  Constant2 : Constant  Value=0.0
  Constant3 : Constant  Value=trim_pitch
  Demux : Demux  Outputs=3
  Demux1 : Demux  Outputs=3
  flip sign1 : Gain  Gain=r2d  SaturateOnIntegerOverflow=on  OutDataTypeStr=Inherit: Same as input  ParamDataTypeStr=Inherit: Same as input
  flip sign3 : Gain  Gain=r2d  SaturateOnIntegerOverflow=on  OutDataTypeStr=Inherit: Same as input  ParamDataTypeStr=Inherit: Same as input
  ic : Subsystem
  ic1 : Subsystem
  ic2 : Subsystem
  ic3 : Subsystem
  phi : Outport  VectorParamsAs1DForOutWhenUnconnected=off
  theta : Outport  Port=2  VectorParamsAs1DForOutWhenUnconnected=off
  psi : Outport  Port=3  VectorParamsAs1DForOutWhenUnconnected=off
  p : Outport  Port=4  VectorParamsAs1DForOutWhenUnconnected=off
  q : Outport  Port=5  VectorParamsAs1DForOutWhenUnconnected=off
  r : Outport  Port=6  VectorParamsAs1DForOutWhenUnconnected=off
  wires:
  Demux1/2 -> ic2/1(u)
  Bus Selector/1 -> flip sign3/1  "<phi_theta_psi>"
  ic/1(y) -> Demux/1
  Bus Selector/2 -> flip sign1/1  "<pqr>"
  Demux/2 -> q/1  "q"
  Constant3/1 -> ic2/2(ic)
  ic1/1(y) -> psi/1  "psi"
  Demux/3 -> r/1  "r"
  flip sign3/1 -> Demux1/1
  ic2/1(y) -> theta/1  "theta"
  Constant2/1 -> ic3/2(ic)
  Constant1/1 -> ic1/2(ic)
  Constant/1 -> ic/2(ic)
  ic3/1(y) -> phi/1  "phi"
  Demux/1 -> p/1  "p"
  AC Bus/1 -> Bus Selector/1
  Demux1/3 -> ic1/1(u)
  flip sign1/1 -> ic/1(u)
  Demux1/1 -> ic3/1(u)

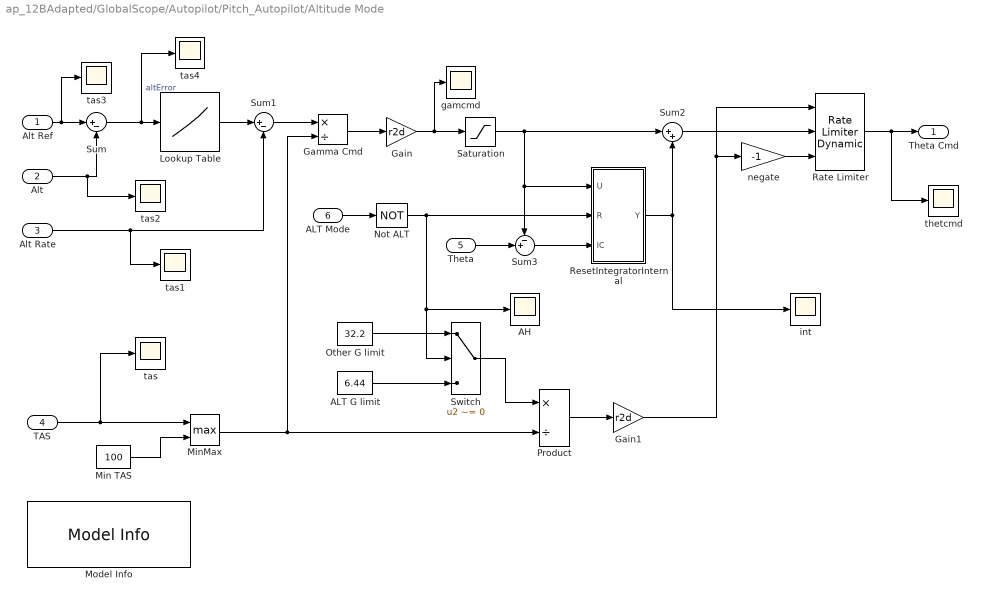
== system ap_12BAdapted/GlobalScope/Autopilot/Pitch_Autopilot/Altitude Mode ==
  Alt Ref : Inport  OutDataTypeStr=double  PortDimensions=1  SampleTime=1/40  Interpolate=off
  Alt : Inport  Port=2  OutDataTypeStr=double  PortDimensions=1  SampleTime=1/40  Interpolate=off
  Alt Rate : Inport  Port=3  OutDataTypeStr=double  PortDimensions=1  SampleTime=1/40  Interpolate=off
  TAS : Inport  Port=4  OutDataTypeStr=double  PortDimensions=1  SampleTime=1/40  Interpolate=off
  Theta : Inport  Port=5  OutDataTypeStr=double  PortDimensions=1  SampleTime=1/40  Interpolate=off
  ALT Mode : Inport  Port=6  OutDataTypeStr=boolean  PortDimensions=1  SampleTime=1/40  Interpolate=off
  AH : Scope
  ALT G limit : Constant  Value=6.44  OutDataTypeStr=double
  Gain : Gain  Gain=r2d
  Gain1 : Gain  Gain=r2d
  Gamma Cmd : Product  Inputs=*/  RndMeth=Zero
  Lookup Table : Lookup_n-D  NumberOfTableDimensions=1  BreakpointsForDimension1=[-544 -206 -116 -52 0 52 116 206]  Table=[-42 -26 -19 -13 0 13 19 26]  ExtrapMethod=Clip  RemoveProtectionInput=on  UseLastTableValue=on  RndMeth=Zero  FractionDataTypeStr=double  InputSameDT=on
  Min TAS : Constant  Value=100  OutDataTypeStr=double
  MinMax : MinMax  Function=max  Inputs=2  InputSameDT=on
  Model Info : simulink/Model-Wide Utilities/Model Info  Frame=on  DisplayStringWithTags=|  HorizontalTextAlignment=Left  LeftAlignmentValue=0.02
      | Altitude Mode
      | Author: %<LastModifiedBy>
      | Version: %<ModelVersion>
      | Date: %<LastModificationDate>
  Not ALT : Logic  Operator=NOT  IconShape=distinctive  AllPortsSameDT=off  OutDataTypeStr=boolean
  Other G limit : Constant  Value=32.2  OutDataTypeStr=double
  Product : Product  Inputs=*/  RndMeth=Zero
  Rate Limiter : simulink/Discontinuities/Rate Limiter Dynamic
      settings: SourceProductName=Simulink
  ResetIntegratorInternal : Subsystem
  Saturation : Saturate  UpperLimit=20  LowerLimit=-20
  Sum : Sum  Inputs=|+-
  Sum1 : Sum  Inputs=|+-
  Sum2 : Sum  Inputs=|++
  Sum3 : Sum  Inputs=-+|
  Switch : Switch  Criteria=u2 ~= 0
  gamcmd : Scope
  int : Scope
  negate : Gain  Gain=-1
  tas{,1..4} (5 alike) : Scope
  thetcmd : Scope
  Theta Cmd : Outport  OutDataTypeStr=double  PortDimensions=1  SampleTime=1/40  VectorParamsAs1DForOutWhenUnconnected=off
  wires:
  Other G limit/1 -> Switch/1
  Alt Ref/1 -> tas3/1, Sum/1
  Min TAS/1 -> MinMax/2
  Lookup Table/1 -> Sum1/1
  Rate Limiter/1 -> thetcmd/1, Theta Cmd/1
  negate/1 -> Rate Limiter/3
  MinMax/1 -> Gamma Cmd/2, Product/2
  Product/1 -> Gain1/1
  Gain1/1 -> negate/1, Rate Limiter/1
  Switch/1 -> Product/1
  ResetIntegratorInternal/1(Y) -> int/1, Sum2/2
  ALT G limit/1 -> Switch/3
  Sum2/1 -> Rate Limiter/2
  Theta/1 -> Sum3/2
  Sum/1 -> tas4/1, Lookup Table/1  "altError"
  Saturation/1 -> Sum3/1, ResetIntegratorInternal/1(U), Sum2/1
  ALT Mode/1 -> Not ALT/1
  Gain/1 -> gamcmd/1, Saturation/1
  Alt/1 -> tas2/1, Sum/2
  Sum1/1 -> Gamma Cmd/1
  Alt Rate/1 -> tas1/1, Sum1/2
  Gamma Cmd/1 -> Gain/1
  Not ALT/1 -> AH/1, Switch/2, ResetIntegratorInternal/2(R)
  Sum3/1 -> ResetIntegratorInternal/3(IC)
  TAS/1 -> tas/1, MinMax/1

== system ap_12BAdapted/GlobalScope/Autopilot/Pitch_Autopilot/Basic Pitch Mode ==
  note: Attitude Control using displacement, rate and integral
  Disp_Cmd : Inport  OutDataTypeStr=double  PortDimensions=1  SampleTime=1/40
  "Disp_FB " : Inport  Port=2  OutDataTypeStr=double  PortDimensions=1  SampleTime=1/40
  Rate_FB : Inport  Port=3  OutDataTypeStr=double  PortDimensions=1  SampleTime=1/40
  Engaged : Inport  Port=4  OutDataTypeStr=boolean  PortDimensions=1  SampleTime=1/40
  Cmd Limit : Saturate  UpperLimit=20  LowerLimit=-20
      settings: AttributesFormatString=%<LowerLimit> to %<UpperLimit> (deg)
  Disp Gain : Gain  Gain=2.0
  Disp Limit : Saturate  UpperLimit=20  LowerLimit=-20
      settings: AttributesFormatString=%<LowerLimit> to %<UpperLimit> (deg)
  Int Gain : Gain  Gain=0.5
  Model Info : simulink/Model-Wide Utilities/Model Info  Frame=on  DisplayStringWithTags=|  HorizontalTextAlignment=Left  LeftAlignmentValue=0.02
      | Attitude Controller
      | Author: %<LastModifiedBy>
      | Version: %<ModelVersion>
      | Date: %<LastModificationDate>
  Not engaged : Logic  Operator=NOT  IconShape=distinctive  AllPortsSameDT=off  OutDataTypeStr=boolean
  Rate Gain : Gain  Gain=2.0
  Rate Limit : Saturate  UpperLimit=3  LowerLimit=-3
      settings: AttributesFormatString=%<LowerLimit> to %<UpperLimit> (deg/sec)
  ResetIntegratorInternal : Subsystem
  Sum : Sum  Inputs=|+-
  Sum1 : Sum  Inputs=|+-
  Sum2 : Sum  Inputs=++|
  att : Scope
  q : Scope
  thet : Scope
  Surf_Cmd : Outport  OutDataTypeStr=double  PortDimensions=1  SampleTime=1/40  VectorParamsAs1DForOutWhenUnconnected=off
  wires:
  Rate Limit/1 -> Sum1/1
  ResetIntegratorInternal/1(Y) -> Sum2/1, att/1
  Sum2/1 -> Cmd Limit/1
  Disp Limit/1 -> Sum/1
  Engaged/1 -> Not engaged/1
  Cmd Limit/1 -> Surf_Cmd/1
  Disp_Cmd/1 -> Disp Limit/1
  Rate_FB/1 -> q/1, Sum1/2
  Sum1/1 -> Rate Gain/1, Int Gain/1
  Sum/1 -> Disp Gain/1
  Disp Gain/1 -> Rate Limit/1
  Rate Gain/1 -> Sum2/2
  "Disp_FB "/1 -> thet/1, Sum/2
  Not engaged/1 -> ResetIntegratorInternal/2(R)
  Int Gain/1 -> ResetIntegratorInternal/1(U)

== system ap_12BAdapted/GlobalScope/Autopilot/Pitch_Autopilot/Pitch Rate Feedback ==
  note: Pitch Rate Computation
  Phi : Inport
  Q : Inport  Port=2
  R : Inport  Port=3
  Gain : Gain  Gain=d2r
  Product : Product  RndMeth=Zero
  Product1 : Product  RndMeth=Zero
  Sum3 : Sum  Inputs=|++
  cos : Trigonometry  Operator=cos  OutputSignalType=real
  q : Scope
  sin : Trigonometry  OutputSignalType=real
  Pitch Rate : Outport  VectorParamsAs1DForOutWhenUnconnected=off
  wires:
  Phi/1 -> Gain/1
  Product/1 -> Sum3/2
  sin/1 -> Product/1
  R/1 -> Product/2
  Gain/1 -> sin/1, cos/1
  Product1/1 -> Sum3/1
  cos/1 -> Product1/1
  Q/1 -> Product1/2
  Sum3/1 -> q/1, Pitch Rate/1

== system ap_12BAdapted/GlobalScope/Autopilot/Pitch_Autopilot/Pitch Reference ==
  note: Pitch Reference
  Theta : Inport
  AP Eng : Inport  Port=2
  Pitch Wheel : Inport  Port=3
  Not engaged : Logic  Operator=NOT  IconShape=distinctive  AllPortsSameDT=off  OutDataTypeStr=boolean
  Sum3 : Sum  Inputs=|++
  latch : Subsystem
  Theta Ref : Outport  VectorParamsAs1DForOutWhenUnconnected=off
  wires:
  Not engaged/1 -> latch/2(E)
  latch/1(y) -> Sum3/1
  Theta/1 -> latch/1(u)
  AP Eng/1 -> Not engaged/1
  Sum3/1 -> Theta Ref/1
  Pitch Wheel/1 -> Sum3/2

== system ap_12BAdapted/GlobalScope/Autopilot/Roll_Autopilot/Basic Roll Mode ==
  note: Attitude Control using displacement, rate and integral
  Disp_Cmd : Inport  OutDataTypeStr=double  PortDimensions=1
  "Disp_FB " : Inport  Port=2  OutDataTypeStr=double  PortDimensions=1  SampleTime=1/40
  Rate_FB : Inport  Port=3  OutDataTypeStr=double  PortDimensions=1  SampleTime=1/40
  Engaged : Inport  Port=4  OutDataTypeStr=boolean  PortDimensions=1  SampleTime=1/40
  Cmd Limit : Saturate  UpperLimit=15  LowerLimit=-15
      settings: AttributesFormatString=%<LowerLimit> to %<UpperLimit> (deg)
  Disp Gain : Gain  Gain=1.0
  Disp Limit : Saturate  UpperLimit=30  LowerLimit=-30
      settings: AttributesFormatString=%<LowerLimit> to %<UpperLimit> (deg)
  Int Gain : Gain  Gain=1.0
  Model Info : simulink/Model-Wide Utilities/Model Info  Frame=on  DisplayStringWithTags=|  HorizontalTextAlignment=Left  LeftAlignmentValue=0.02
      | Attitude Controller
      | Author: %<LastModifiedBy>
      | Version: %<ModelVersion>
      | Date: %<LastModificationDate>
  Not engaged : Logic  Operator=NOT  IconShape=distinctive  AllPortsSameDT=off  OutDataTypeStr=boolean
  Rate Gain : Gain  Gain=3.0
  Rate Limit : Saturate  UpperLimit=6  LowerLimit=-6
      settings: AttributesFormatString=%<LowerLimit> to %<UpperLimit> (deg/sec)
  ResetIntegratorInternal : Subsystem
  Scope : Scope
  Scope1 : Scope
  Scope2 : Scope
  Sum : Sum  Inputs=|+-
  Sum1 : Sum  Inputs=|+-
  Sum2 : Sum  Inputs=++|
  Surf_Cmd : Outport  OutDataTypeStr=double  PortDimensions=1  SampleTime=1/40  VectorParamsAs1DForOutWhenUnconnected=off
  wires:
  Engaged/1 -> Not engaged/1
  Disp_Cmd/1 -> Disp Limit/1
  Rate Limit/1 -> Sum1/1
  ResetIntegratorInternal/1(Y) -> Sum2/1, Scope/1
  Not engaged/1 -> ResetIntegratorInternal/2(R)
  Rate_FB/1 -> Sum1/2
  Sum1/1 -> Int Gain/1, Scope1/1, Rate Gain/1
  Cmd Limit/1 -> Scope2/1, Surf_Cmd/1
  Rate Gain/1 -> Sum2/2
  Disp Gain/1 -> Rate Limit/1
  Sum/1 -> Disp Gain/1
  "Disp_FB "/1 -> Sum/2
  Disp Limit/1 -> Sum/1
  Sum2/1 -> Cmd Limit/1
  Int Gain/1 -> ResetIntegratorInternal/1(U)

== system ap_12BAdapted/GlobalScope/Autopilot/Roll_Autopilot/Heading Mode ==
  Psi Ref : Inport  OutDataTypeStr=double  PortDimensions=1  SampleTime=1/40  Interpolate=off
  Psi : Inport  Port=2  OutDataTypeStr=double  PortDimensions=1  SampleTime=1/40  Interpolate=off
  TAS : Inport  Port=3  OutDataTypeStr=double  PortDimensions=1  SampleTime=1/40  Interpolate=off
  Disp Gain : Gain  Gain=0.015
  Model Info : simulink/Model-Wide Utilities/Model Info  Frame=on  DisplayStringWithTags=|  HorizontalTextAlignment=Left  LeftAlignmentValue=0.02
      | Heading Mode
      | Author: %<LastModifiedBy>
      | Version: %<ModelVersion>
      | Date: %<LastModificationDate>
  Product : Product  RndMeth=Zero
  angle diff : Subsystem
  Phi Cmd : Outport  OutDataTypeStr=double  PortDimensions=1  SampleTime=1/40  VectorParamsAs1DForOutWhenUnconnected=off
  wires:
  Psi Ref/1 -> angle diff/1(plus)
  angle diff/1(diff) -> Disp Gain/1  "hdgError"
  TAS/1 -> Product/2
  Disp Gain/1 -> Product/1
  Psi/1 -> angle diff/2(minus)
  Product/1 -> Phi Cmd/1

== system ap_12BAdapted/GlobalScope/Autopilot/Roll_Autopilot/Roll Reference ==
  note: Roll Reference
  Phi : Inport
  AP eng : Inport  Port=2
  Turn Knob : Inport  Port=3
  Abs : Abs
  Not engaged : Logic  Operator=NOT  IconShape=distinctive  AllPortsSameDT=off  OutDataTypeStr=boolean
  Ref Threshold : RelationalOperator  OutDataTypeStr=boolean  RndMeth=Nearest  InputSameDT=on
  Ref Threshold1 : RelationalOperator  Operator=<=  OutDataTypeStr=boolean  RndMeth=Nearest  InputSameDT=on
  TK Threshold : RelationalOperator  Operator=<  OutDataTypeStr=boolean  RndMeth=Nearest  InputSameDT=on
  TK switch : Switch  Criteria=u2 ~= 0
  latch : Subsystem
  minus six : Constant  Value=-6
  or : Logic  Operator=OR  IconShape=distinctive  OutDataTypeStr=boolean
  ref switch : Switch  Criteria=u2 ~= 0
  six : Constant  Value=6
  three : Constant  Value=3  OutDataTypeStr=double
  zero : Constant  Value=0
  Phi Ref : Outport  VectorParamsAs1DForOutWhenUnconnected=off
  wires:
  minus six/1 -> Ref Threshold1/2
  Ref Threshold1/1 -> or/2
  Ref Threshold/1 -> or/1
  or/1 -> ref switch/2
  zero/1 -> ref switch/3
  six/1 -> Ref Threshold/2
  TK switch/1 -> Phi Ref/1
  AP eng/1 -> Not engaged/1
  Phi/1 -> Ref Threshold1/1, Ref Threshold/1, ref switch/1
  Abs/1 -> TK Threshold/1
  three/1 -> TK Threshold/2
  Turn Knob/1 -> Abs/1, TK switch/3
  TK Threshold/1 -> TK switch/2
  latch/1(y) -> TK switch/1
  ref switch/1 -> latch/1(u)
  Not engaged/1 -> latch/2(E)

== system ap_12BAdapted/GlobalScope/Autopilot/Yaw_damper/Basic Yaw Damper ==
  note: Basic Yaw Damper
  "Phi " : Inport
  R : Inport  Port=2
  TAS : Inport  Port=3
  Constant : Constant  Value=100
  MinMax : MinMax  Function=max  Inputs=2
  Model Info : simulink/Model-Wide Utilities/Model Info  Frame=on  DisplayStringWithTags=|  HorizontalTextAlignment=Left  LeftAlignmentValue=0.02
      | Yaw Damper
      | Author: %<LastModifiedBy>
      | Date: %<LastModificationDate>
      | Model Version: %<ModelVersion>
  Product : Product  Inputs=*/  RndMeth=Zero
  Rate Gain : Gain  Gain=1.0
  Rud Limit : Saturate  UpperLimit=25  LowerLimit=-25
      settings: AttributesFormatString=%<LowerLimit> to %<UpperLimit> (deg)
  Sum1 : Sum  Inputs=|+-
  gravity : Gain  Gain=32.2
  sin : Trigonometry
  Rud Cmd : Outport  VectorParamsAs1DForOutWhenUnconnected=off
  wires:
  R/1 -> Sum1/2
  Sum1/1 -> Rate Gain/1  "yawRate"
  Rud Limit/1 -> Rud Cmd/1
  Rate Gain/1 -> Rud Limit/1
  "Phi "/1 -> sin/1
  sin/1 -> gravity/1
  Product/1 -> Sum1/1
  gravity/1 -> Product/1
  MinMax/1 -> Product/2
  TAS/1 -> MinMax/1
  Constant/1 -> MinMax/2

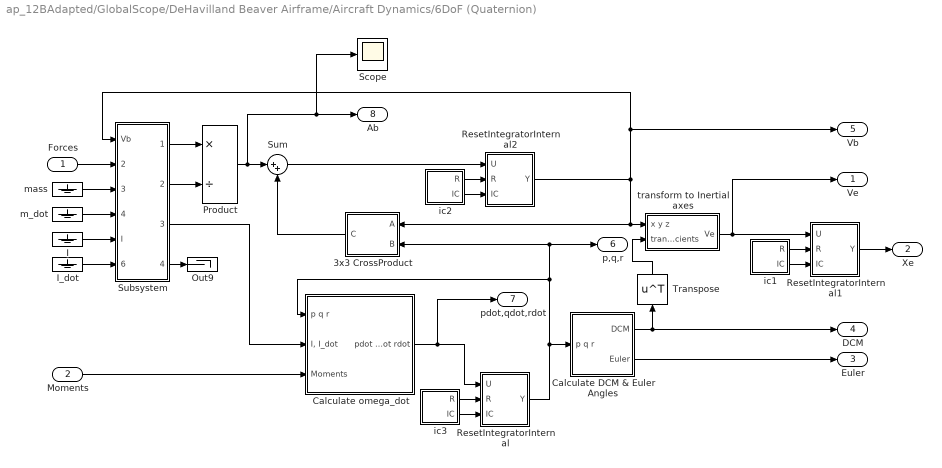
== system ap_12BAdapted/GlobalScope/DeHavilland Beaver Airframe/Aircraft Dynamics/6DoF (Quaternion) ==
  Forces : Inport
  Moments : Inport  Port=2
  3x3 CrossProduct : Subsystem
  Calculate DCM & Euler Angles : Subsystem
  Calculate omega_dot : Subsystem
  I : Ground
  I_dot : Ground
  Out9 : Terminator
  Product : Product  Inputs=*/  SaturateOnIntegerOverflow=on  OutDataTypeStr=Inherit: Same as first input
  ResetIntegratorInternal : Subsystem
  ResetIntegratorInternal1 : Subsystem
  ResetIntegratorInternal2 : Subsystem
  Scope : Scope
  Subsystem : Subsystem
  Sum : Sum  Inputs=|++  SaturateOnIntegerOverflow=on
  Transpose : Math  Operator=transpose  SaturateOnIntegerOverflow=on
  ic1 : Subsystem
  ic2 : Subsystem
  ic3 : Subsystem
  m_dot : Ground
  mass : Ground
  "transform to Inertial axes " : Subsystem
  Ve : Outport  VectorParamsAs1DForOutWhenUnconnected=off
  Xe : Outport  Port=2  VectorParamsAs1DForOutWhenUnconnected=off
  Euler : Outport  Port=3  VectorParamsAs1DForOutWhenUnconnected=off
  DCM : Outport  Port=4  VectorParamsAs1DForOutWhenUnconnected=off
  Vb : Outport  Port=5  VectorParamsAs1DForOutWhenUnconnected=off
  p,q,r : Outport  Port=6  VectorParamsAs1DForOutWhenUnconnected=off
  pdot,qdot,rdot : Outport  Port=7  VectorParamsAs1DForOutWhenUnconnected=off
  Ab : Outport  Port=8  VectorParamsAs1DForOutWhenUnconnected=off
  wires:
  Subsystem/1("forces ") -> Product/1
  I_dot/1 -> Subsystem/6(I_dot)
  I/1 -> Subsystem/5(I)
  Calculate omega_dot/1(pdot qdot rdot) -> pdot,qdot,rdot/1, ResetIntegratorInternal/1(U)
  Subsystem/4(Out9) -> Out9/1
  m_dot/1 -> Subsystem/4(m_dot)
  Subsystem/2(mass) -> Product/2
  mass/1 -> Subsystem/3("mass ")
  Transpose/1 -> "transform to Inertial axes "/2(transform coefficients)
  Calculate DCM & Euler Angles/1(DCM) -> DCM/1, Transpose/1
  Product/1 -> Scope/1, Ab/1, Sum/1
  Forces/1 -> Subsystem/2(forces)
  Moments/1 -> Calculate omega_dot/3(Moments)
  ResetIntegratorInternal1/1(Y) -> Xe/1
  Sum/1 -> ResetIntegratorInternal2/1(U)
  3x3 CrossProduct/1(C) -> Sum/2
  Calculate DCM & Euler Angles/2(Euler) -> Euler/1
  Subsystem/3("inertia, 0") -> Calculate omega_dot/2("I, I_dot")
  "transform to Inertial axes "/1(Ve) -> ResetIntegratorInternal1/1(U), Ve/1
  ResetIntegratorInternal/1(Y) -> Calculate DCM & Euler Angles/1(p q r), 3x3 CrossProduct/2(B), p,q,r/1, Calculate omega_dot/1(p q r)
  ic3/1(R) -> ResetIntegratorInternal/2(R)
  ic3/2(IC) -> ResetIntegratorInternal/3(IC)
  ic1/1(R) -> ResetIntegratorInternal1/2(R)
  ic1/2(IC) -> ResetIntegratorInternal1/3(IC)
  ic2/1(R) -> ResetIntegratorInternal2/2(R)
  ic2/2(IC) -> ResetIntegratorInternal2/3(IC)
  ResetIntegratorInternal2/1(Y) -> Subsystem/1(Vb), Vb/1, 3x3 CrossProduct/1(A), "transform to Inertial axes "/1(x y z)

== system ap_12BAdapted/GlobalScope/DeHavilland Beaver Airframe/Aircraft Dynamics/Total Forces and Moments ==
  EnvirBus : Inport
  Pilot : Inport  Port=2
  DCM : Inport  Port=3
  FltParams : Inport  Port=4
  Actuators : Subsystem
  Aerodynamics : Subsystem
  Bus Selector4 : BusSelector  OutputSignals=rho,g
  "Engine " : Subsystem
  Forces and Moments : Subsystem
  "Gravity " : Subsystem
  "Pilot " : InportShadow  Port=2
  Sum : Sum  Inputs=|++  SaturateOnIntegerOverflow=on  InputSameDT=on  OutDataTypeStr=Inherit: Same as first input
  Total Force : Outport  VectorParamsAs1DForOutWhenUnconnected=off
  Total Moment : Outport  Port=2  VectorParamsAs1DForOutWhenUnconnected=off
  wires:
  Forces and Moments/1(XYZ) -> Sum/1
  "Engine "/1(Engine Coefficients) -> Forces and Moments/3(Engine Coefficients)
  "Gravity "/1(Fgrav) -> Sum/2
  Aerodynamics/1(Aero Coefficients) -> Forces and Moments/1(Aero Coefficients)
  Pilot/1 -> Actuators/1(Pilot)
  Bus Selector4/1 -> "Engine "/3(rho)  "<rho>"
  DCM/1 -> "Gravity "/2(DCM)
  Bus Selector4/2 -> "Gravity "/1(g)  "<g>"
  Sum/1 -> Total Force/1  "Ftot"
  Forces and Moments/2(LMN) -> Total Moment/1  "Mtot"
  "Pilot "/1 -> "Engine "/2(Pilot)
  FltParams/1 -> Forces and Moments/2(Fltparams), "Engine "/1(Fltparams), Aerodynamics/2(FltParams)
  Actuators/1(uaero-out) -> Aerodynamics/1(Uaero)
  EnvirBus/1 -> Bus Selector4/1

== system ap_12BAdapted/GlobalScope/DeHavilland Beaver Airframe/Calculate Parameters/ Incidence, Sideslip, & Airspeed ==
  Vb : Inport
  Airspeed : Sqrt  AlgorithmType=Newton-Raphson  SaturateOnIntegerOverflow=on
  Incidence : Trigonometry  Operator=atan2
  Product : Product  Inputs=*/  SaturateOnIntegerOverflow=on  OutDataTypeStr=Inherit: Same as first input
  Sideslip : Trigonometry  Operator=asin
  Subsystem : Subsystem
  Subsystem1 : Subsystem
  dot : Subsystem
  Alpha : Outport  VectorParamsAs1DForOutWhenUnconnected=off
  Beta : Outport  Port=2  VectorParamsAs1DForOutWhenUnconnected=off
  V : Outport  Port=3  VectorParamsAs1DForOutWhenUnconnected=off
  wires:
  Sideslip/1 -> Beta/1
  Subsystem1/1(v) -> Product/1
  Product/1 -> Sideslip/1
  Subsystem/1(w) -> Incidence/1
  Subsystem/2(U) -> Incidence/2
  dot/1(dot) -> Airspeed/1
  Airspeed/1 -> V/1, Product/2
  Incidence/1 -> Alpha/1
  Vb/1 -> Subsystem/1(V), dot/1(Vb), Subsystem1/1(V)

== system ap_12BAdapted/GlobalScope/DeHavilland Beaver Airframe/Calculate Parameters/Dynamic Pressure ==
  Velocity : Inport
  Air Density : Inport  Port=2
  1/2rhoV^2 : Gain  Gain=0.5  SaturateOnIntegerOverflow=on  OutDataTypeStr=Inherit: Same as input  ParamDataTypeStr=Inherit: Same as input
  Product2 : Product  SaturateOnIntegerOverflow=on  InputSameDT=on  OutDataTypeStr=Inherit: Same as first input
  dot : Subsystem
  qbar : Outport  VectorParamsAs1DForOutWhenUnconnected=off
  wires:
  1/2rhoV^2/1 -> qbar/1
  Air Density/1 -> Product2/2
  dot/1(dot) -> Product2/1
  Product2/1 -> 1/2rhoV^2/1
  Velocity/1 -> dot/1(V)

== system ap_12BAdapted/GlobalScope/Sensors/Air Data Sensor/ Incidence, Sideslip, & Airspeed ==
  Vb : Inport
  Airspeed : Sqrt  AlgorithmType=Newton-Raphson  SaturateOnIntegerOverflow=on
  Gain : Gain  Gain=180/pi
  Gain1 : Gain  Gain=180/pi
  Incidence : Trigonometry  Operator=atan2
  Product : Product  Inputs=*/  SaturateOnIntegerOverflow=on  OutDataTypeStr=Inherit: Same as first input
  Scope : Scope
  Scope1 : Scope
  Sideslip : Trigonometry  Operator=asin
  Subsystem : Subsystem
  Subsystem1 : Subsystem
  dot : Subsystem
  Alpha : Outport  VectorParamsAs1DForOutWhenUnconnected=off
  Beta : Outport  Port=2  VectorParamsAs1DForOutWhenUnconnected=off
  V : Outport  Port=3  VectorParamsAs1DForOutWhenUnconnected=off
  wires:
  Sideslip/1 -> Gain1/1, Beta/1
  Subsystem1/1(v) -> Product/1
  Product/1 -> Sideslip/1
  Subsystem/1(w) -> Incidence/1
  Subsystem/2(U) -> Incidence/2
  dot/1(dot) -> Airspeed/1
  Airspeed/1 -> V/1, Product/2
  Incidence/1 -> Gain/1, Alpha/1
  Vb/1 -> Subsystem/1(V), dot/1(Vb), Subsystem1/1(V)
  Gain/1 -> Scope/1
  Gain1/1 -> Scope1/1

== system ap_12BAdapted/GlobalScope/Sensors/Air Data Sensor/ic1 ==
  u : Inport
  ic : Inport  Port=2
  Constant : Constant
  Switch : Switch  Criteria=u2 ~= 0
  Unit Delay : UnitDelay  SampleTime=-1  HasFrameUpgradeWarning=on
  y : Outport  VectorParamsAs1DForOutWhenUnconnected=off
  wires:
  Switch/1 -> y/1
  u/1 -> Switch/1
  ic/1 -> Switch/3
  Constant/1 -> Unit Delay/1
  Unit Delay/1 -> Switch/2

== system ap_12BAdapted/GlobalScope/Sensors/Air Data Sensor/ic2 ==
  u : Inport
  ic : Inport  Port=2
  Constant : Constant
  Switch : Switch  Criteria=u2 ~= 0
  Unit Delay : UnitDelay  SampleTime=-1  HasFrameUpgradeWarning=on
  y : Outport  VectorParamsAs1DForOutWhenUnconnected=off
  wires:
  ic/1 -> Switch/3
  u/1 -> Switch/1
  Switch/1 -> y/1
  Constant/1 -> Unit Delay/1
  Unit Delay/1 -> Switch/2

== system ap_12BAdapted/GlobalScope/Sensors/Air Data Sensor/ic3 ==
  u : Inport
  ic : Inport  Port=2
  Constant1 : Constant
  Switch : Switch  Criteria=u2 ~= 0
  Unit Delay1 : UnitDelay  SampleTime=-1  HasFrameUpgradeWarning=on
  y : Outport  VectorParamsAs1DForOutWhenUnconnected=off
  wires:
  ic/1 -> Switch/3
  u/1 -> Switch/1
  Switch/1 -> y/1
  Constant1/1 -> Unit Delay1/1
  Unit Delay1/1 -> Switch/2

== system ap_12BAdapted/GlobalScope/Sensors/Inertial Data Sensor/ic ==
  u : Inport
  ic : Inport  Port=2
  Constant : Constant
  Switch : Switch  Criteria=u2 ~= 0
  Unit Delay : UnitDelay  SampleTime=-1  HasFrameUpgradeWarning=on
  y : Outport  VectorParamsAs1DForOutWhenUnconnected=off
  wires:
  Switch/1 -> y/1
  u/1 -> Switch/1
  ic/1 -> Switch/3
  Constant/1 -> Unit Delay/1
  Unit Delay/1 -> Switch/2

== system ap_12BAdapted/GlobalScope/Sensors/Inertial Data Sensor/ic1 ==
  u : Inport
  ic : Inport  Port=2
  Constant : Constant
  Switch : Switch  Criteria=u2 ~= 0
  Unit Delay : UnitDelay  SampleTime=-1  HasFrameUpgradeWarning=on
  y : Outport  VectorParamsAs1DForOutWhenUnconnected=off
  wires:
  ic/1 -> Switch/3
  u/1 -> Switch/1
  Switch/1 -> y/1
  Constant/1 -> Unit Delay/1
  Unit Delay/1 -> Switch/2

== system ap_12BAdapted/GlobalScope/Sensors/Inertial Data Sensor/ic2 ==
  u : Inport
  ic : Inport  Port=2
  Constant : Constant
  Switch : Switch  Criteria=u2 ~= 0
  Unit Delay : UnitDelay  SampleTime=-1  HasFrameUpgradeWarning=on
  y : Outport  VectorParamsAs1DForOutWhenUnconnected=off
  wires:
  Switch/1 -> y/1
  u/1 -> Switch/1
  ic/1 -> Switch/3
  Constant/1 -> Unit Delay/1
  Unit Delay/1 -> Switch/2
